simulink model "ulise_internal_v0"  (R2025b)
settings: Solver=FixedStepAuto  StartTime=0.0  StopTime=SimSetup.K - 1  FixedStep=1  RelTol=1e-3
InitFcn:
  | InitFcn_ULISE
model workspace (MAT data in the model file):
  Something = 3
undefined symbols (not defined in the file): A, B, C, D, G, H, Q, R, Sigma, SimSetup, U1, U2, V, V1, V2, x0
libraries: dspinverses x1
settings Model: Creator=savan  LastModifiedBy=daniellawson
settings DebuggingCC: AlgebraicLoopMsg=none

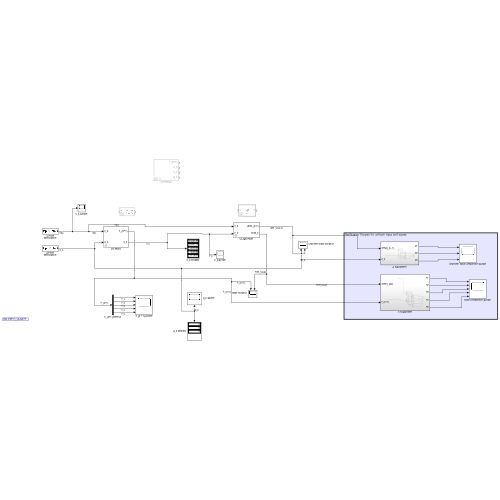
[thumbnail: Simulink's stored preview of the top-level diagram]
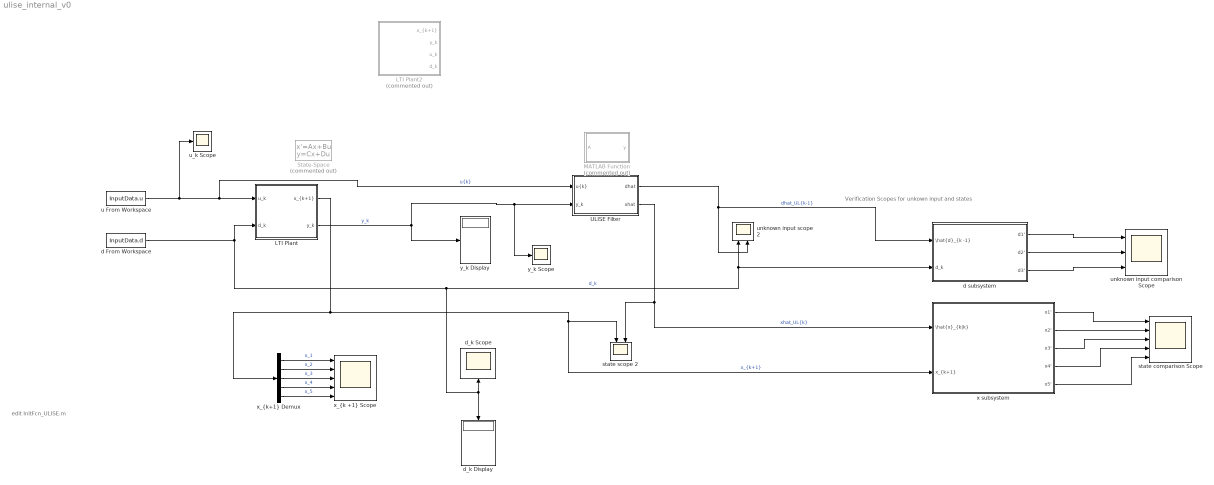
== system ulise_internal_v0 ==
  note: edit InitFcn_ULISE.m
  note: Verification Scopes for unkown input and states
  " u From Workspace" : FromWorkspace  VariableName=InputData.u  SampleTime=SimSetup.Ts  Interpolate=off  OutputAfterFinalValue=Holding final value
  LTI Plant : Subsystem  mask{x0=x0, Ts=SimSetup.Ts}
      mask prompts: x0 "Initial states x[0]:"; Ts "Sample Time (-1 for Inherited):"
      mask help:
      | Simulate the states and measurements of a discrete-time, time-invariant linear system of the form
      |
      | x[k+1] = Ax[k] + Bu[k] + Gd[k]
      | y[k] = Cx[k] + Du[k] + Hd[k].
      mask DialogControl DescGroupVar Prompt: Plant
      mask DialogControl InitialConditions Prompt: Initial Conditions
      mask Display:
      | port_label('input', 1, 'u_k');
      | port_label('input', 2, 'd_k');
      | port_label('output', 1, 'x_{k+1}');
      | port_label('output', 2, 'y_k');
  LTI Plant2 : Subsystem  Commented=on  mask{x0=x0, Ts=SimSetup.Ts}
      mask prompts: x0 "Initial states x[0]:"; Ts "Sample Time (-1 for Inherited):"
      mask help: Simulate the states and measurements of a discrete-time, time-invariant linear system. The user-defined known and unknown inputs are also returned.
      mask DialogControl DescGroupVar Prompt: Plant
      mask DialogControl InitialConditions Prompt: Initial Conditions
      mask Display:
      | port_label('output', 1, 'x_{k+1}');
      | port_label('output', 2, 'y_k');
      | port_label('output', 3, 'u_k');
      | port_label('output', 4, 'd_k');
  MATLAB Function : MATLAB Function  Commented=on  TreatAsAtomicUnit=on
  State-Space : StateSpace  Commented=on  InitialCondition=0
  ULISE Filter : Subsystem  mask{Ts=-1}
      mask prompts: Ts "Sample time (-1 for Inherited):"
      mask help: Estimates the states and unknown inputs of a discrete-time, time-invariant linear system. The states are estimated with a zero-step delay, while the unknown inputs are estimated with a one-step delay.
      mask DialogControl DescGroupVar Prompt: ULISE Filter
      mask Display:
      | port_label('input', 1, 'u_k');
      | port_label('input', 2, 'y_k');
      | port_label('output', 1, 'dhat_{k-1}');
      | port_label('output', 2, 'xhat_k');
  d From Workspace : FromWorkspace  VariableName=InputData.d  SampleTime=SimSetup.Ts  Interpolate=off  OutputAfterFinalValue=Holding final value
  d subsystem : Subsystem
  d_k Display : Display
  d_k Scope : Scope
      settings: ActiveDisplayYMinimum=-3.75  ActiveDisplayYMaximum=3.75
  state comparison Scope : Scope  NumInputPorts=5
      settings: ActiveDisplayString=5  ActiveDisplayYMinimum=-0.034557973978604738  ActiveDisplayYMaximum=0.034947051285830096  YLabel=x_5  DataLoggingVariableName=ScopeData7
  state scope 2 : Scope  NumInputPorts=2
      settings: ActiveDisplayYMinimum=-1  ActiveDisplayYMaximum=1  DataLoggingVariableName=ScopeData9
  u_k Scope : Scope
      settings: ActiveDisplayYMinimum=-0.9712898122759519  ActiveDisplayYMaximum=0.99793476405615489  DataLoggingVariableName=ScopeData2
  unknown input comparison Scope : Scope  NumInputPorts=3
      settings: ActiveDisplayString=3  ActiveDisplayYMinimum=-5.0027563624884559  ActiveDisplayYMaximum=4.879938565566035  YLabel=d_3  DataLoggingVariableName=ScopeData8
  unknown input scope 2 : Scope  NumInputPorts=2
      settings: ActiveDisplayYMinimum=-3.75  ActiveDisplayYMaximum=3.75  DataLoggingVariableName=ScopeData10
  x subsystem : Subsystem
  "x_{k +1} Scope" : Scope  NumInputPorts=5
      settings: Title=%<SignalLabel> vs. time  ActiveDisplayYMinimum=-3.2438704596017818  ActiveDisplayYMaximum=10.248440676542884  YLabel=x_1  DataLoggingVariableName=ScopeData4
  "x_{k+1} Demux" : Demux  Outputs=size(A,1)
  y_k Display : Display
  y_k Scope : Scope
      settings: ActiveDisplayYMinimum=-7.4398331257700985  ActiveDisplayYMaximum=13.958793119448332
  wires:
  x subsystem/1(x1') -> state comparison Scope/1
  x subsystem/2(x2') -> state comparison Scope/2
  x subsystem/3(x3') -> state comparison Scope/3
  x subsystem/4(x4') -> state comparison Scope/4
  x subsystem/5(x5') -> state comparison Scope/5
  d subsystem/1(d1') -> unknown input comparison Scope/1
  d subsystem/2(d2') -> unknown input comparison Scope/2
  d subsystem/3(d3') -> unknown input comparison Scope/3
  ULISE Filter/2(xhat) -> x subsystem/1("\\hat{x}_{k|k}"), state scope 2/2  "xhat_UL{k}"
  ULISE Filter/1(dhat) -> d subsystem/1("\\hat{d}_{k -1}"), unknown input scope 2/2  "dhat_UL{k-1}"
  " u From Workspace"/1 -> u_k Scope/1, LTI Plant/1(u_k), ULISE Filter/1("u{k}")  "u{k}"
  LTI Plant/2(y_k) -> y_k Display/1, y_k Scope/1, ULISE Filter/2(y_k)  "y_k"
  "x_{k+1} Demux"/1 -> "x_{k +1} Scope"/1  "x_1"
  "x_{k+1} Demux"/2 -> "x_{k +1} Scope"/2  "x_2"
  "x_{k+1} Demux"/4 -> "x_{k +1} Scope"/4  "x_4"
  "x_{k+1} Demux"/3 -> "x_{k +1} Scope"/3  "x_3"
  "x_{k+1} Demux"/5 -> "x_{k +1} Scope"/5  "x_5"
  LTI Plant/1("x_{k+1}") -> "x_{k+1} Demux"/1, x subsystem/2("x_{k+1}"), state scope 2/1  "x_{k+1}"
  d From Workspace/1 -> d_k Scope/1, d_k Display/1, d subsystem/2(d_k), unknown input scope 2/1, LTI Plant/2(d_k)  "d_k"

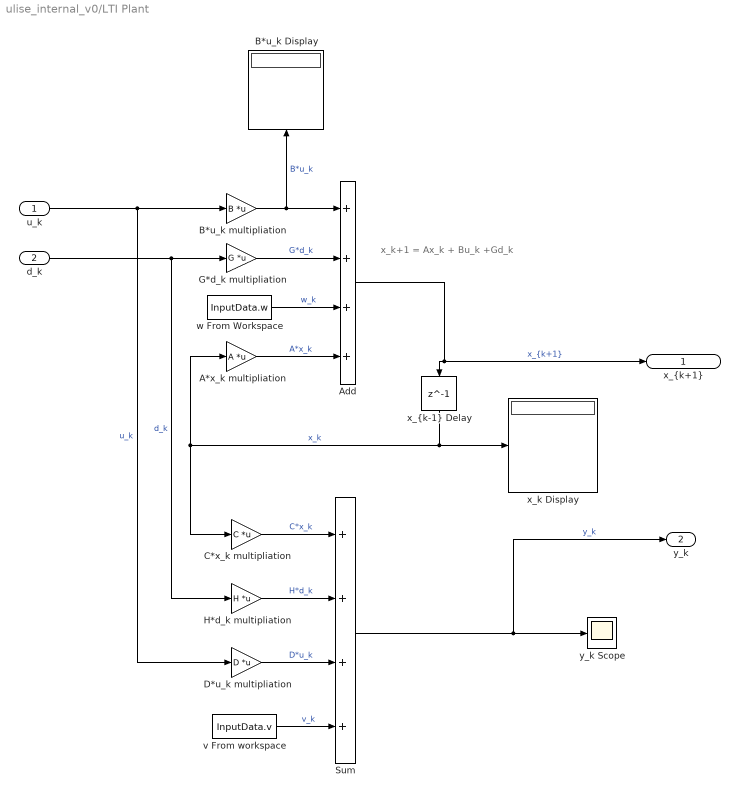
== system ulise_internal_v0/LTI Plant ==
  note: x_k+1 = Ax_k + Bu_k +Gd_k
  u_k : Inport
  d_k : Inport  Port=2
  A*x_k multipliation : Gain  Gain=A  Multiplication=Matrix(K*u)
  Add : Sum  Inputs=++++
  B*u_k Display : Display
  B*u_k multipliation : Gain  Gain=B  Multiplication=Matrix(K*u)
  C*x_k multipliation : Gain  Gain=C  Multiplication=Matrix(K*u)
  D*u_k multipliation : Gain  Gain=D  Multiplication=Matrix(K*u)
  G*d_k multipliation : Gain  Gain=G  Multiplication=Matrix(K*u)
  H*d_k multipliation : Gain  Gain=H  Multiplication=Matrix(K*u)
  Sum : Sum  Inputs=++++
  v From workspace : FromWorkspace  VariableName=InputData.v  SampleTime=SimSetup.Ts  Interpolate=off  OutputAfterFinalValue=Holding final value
  w From Workspace : FromWorkspace  VariableName=InputData.w  SampleTime=SimSetup.Ts  Interpolate=off  OutputAfterFinalValue=Holding final value
  x_k Display : Display
  "x_{k-1} Delay" : Delay  DelayLength=1  InitialCondition=x0
  y_k Scope : Scope
      settings: ActiveDisplayYMinimum=-7.0592065430833646  ActiveDisplayYMaximum=14.061490045979077  DataLoggingVariableName=ScopeData5
  "x_{k+1}" : Outport
  y_k : Outport  Port=2
  wires:
  D*u_k multipliation/1 -> Sum/3  "D*u_k"
  v From workspace/1 -> Sum/4  "v_k"
  H*d_k multipliation/1 -> Sum/2  "H*d_k"
  G*d_k multipliation/1 -> Add/2  "G*d_k"
  C*x_k multipliation/1 -> Sum/1  "C*x_k"
  Sum/1 -> y_k/1, y_k Scope/1  "y_k"
  "x_{k-1} Delay"/1 -> A*x_k multipliation/1, C*x_k multipliation/1, x_k Display/1  "x_k"
  w From Workspace/1 -> Add/3  "w_k"
  B*u_k multipliation/1 -> Add/1, B*u_k Display/1  "B*u_k"
  Add/1 -> "x_{k+1}"/1, "x_{k-1} Delay"/1  "x_{k+1}"
  A*x_k multipliation/1 -> Add/4  "A*x_k"
  d_k/1 -> H*d_k multipliation/1, G*d_k multipliation/1  "d_k"
  u_k/1 -> D*u_k multipliation/1, B*u_k multipliation/1  "u_k"

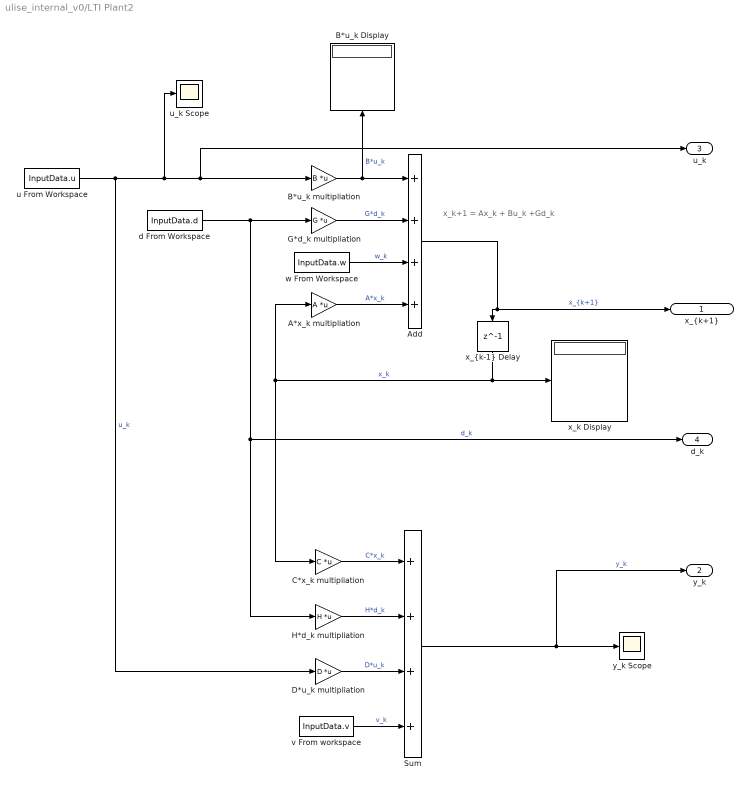
== system ulise_internal_v0/LTI Plant2 ==
  note: x_k+1 = Ax_k + Bu_k +Gd_k
  " u From Workspace" : FromWorkspace  VariableName=InputData.u  SampleTime=SimSetup.Ts  Interpolate=off  OutputAfterFinalValue=Holding final value
  A*x_k multipliation : Gain  Gain=A  Multiplication=Matrix(K*u)
  Add : Sum  Inputs=++++
  B*u_k Display : Display
  B*u_k multipliation : Gain  Gain=B  Multiplication=Matrix(K*u)
  C*x_k multipliation : Gain  Gain=C  Multiplication=Matrix(K*u)
  D*u_k multipliation : Gain  Gain=D  Multiplication=Matrix(K*u)
  G*d_k multipliation : Gain  Gain=G  Multiplication=Matrix(K*u)
  H*d_k multipliation : Gain  Gain=H  Multiplication=Matrix(K*u)
  Sum : Sum  Inputs=++++
  d From Workspace : FromWorkspace  VariableName=InputData.d  SampleTime=SimSetup.Ts  Interpolate=off  OutputAfterFinalValue=Holding final value
  u_k Scope : Scope
      settings: ActiveDisplayYMinimum=-0.9712898122759519  ActiveDisplayYMaximum=0.99793476405615489  DataLoggingVariableName=ScopeData6
  v From workspace : FromWorkspace  VariableName=InputData.v  SampleTime=SimSetup.Ts  Interpolate=off  OutputAfterFinalValue=Holding final value
  w From Workspace : FromWorkspace  VariableName=InputData.w  SampleTime=SimSetup.Ts  Interpolate=off  OutputAfterFinalValue=Holding final value
  x_k Display : Display
  "x_{k-1} Delay" : Delay  DelayLength=1  InitialCondition=x0
  y_k Scope : Scope
      settings: ActiveDisplayYMinimum=-7.0592065430833646  ActiveDisplayYMaximum=14.061490045979077  DataLoggingVariableName=ScopeData5
  "x_{k+1}" : Outport
  y_k : Outport  Port=2
  u_k : Outport  Port=3
  d_k : Outport  Port=4
  wires:
  D*u_k multipliation/1 -> Sum/3  "D*u_k"
  v From workspace/1 -> Sum/4  "v_k"
  " u From Workspace"/1 -> u_k Scope/1, u_k/1, B*u_k multipliation/1, D*u_k multipliation/1  "u_k"
  H*d_k multipliation/1 -> Sum/2  "H*d_k"
  G*d_k multipliation/1 -> Add/2  "G*d_k"
  C*x_k multipliation/1 -> Sum/1  "C*x_k"
  Sum/1 -> y_k/1, y_k Scope/1  "y_k"
  "x_{k-1} Delay"/1 -> A*x_k multipliation/1, C*x_k multipliation/1, x_k Display/1  "x_k"
  w From Workspace/1 -> Add/3  "w_k"
  d From Workspace/1 -> H*d_k multipliation/1, d_k/1, G*d_k multipliation/1  "d_k"
  B*u_k multipliation/1 -> Add/1, B*u_k Display/1  "B*u_k"
  Add/1 -> "x_{k+1}"/1, "x_{k-1} Delay"/1  "x_{k+1}"
  A*x_k multipliation/1 -> Add/4  "A*x_k"

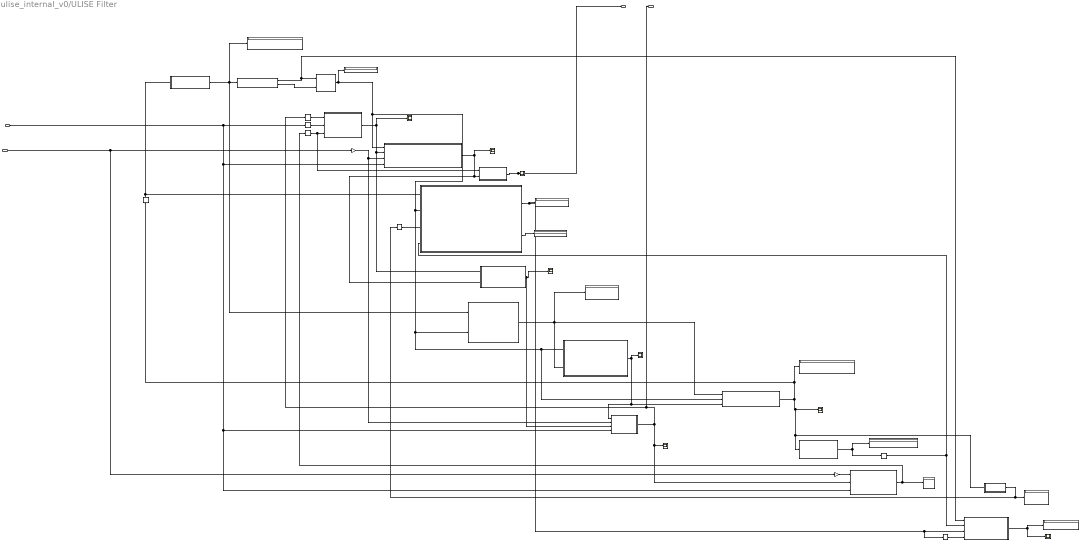
== system ulise_internal_v0/ULISE Filter ==
  note: estimate d1
  "u{k}" : Inport
  y_k : Inport  Port=2
  "Compute L_{k}" : Subsystem
  "Compute M_UL{k}" : Subsystem
  "Compute P_tilde_UL{k}" : Subsystem
  "Compute Pd12_{k-1} and Pxd2_{k-1}" : Subsystem
  "Compute Pd1_{k}" : Subsystem
  "Compute Pd2_{k-1}" : Subsystem
  "Compute Pd_{k -1}" : Subsystem
  "Compute Px_star_{k}" : Subsystem
  "Compute Px_{k | k}" : Subsystem
  "Compute Pxd1_{k}" : Subsystem
  "Compute measurement update, xhat_{k | k}" : Subsystem
  "Compute observable unknown input, dhat1_{k}" : Subsystem
  "Compute state prediction, xhat_{k | k-1} " : Subsystem
  "Compute time updated state, xhat_star_{k | k}" : Subsystem
  "Compute unknown input, dhat_{k-1}" : Subsystem
  "Compute unobservable unknown input, dhat2_{k-1}" : Subsystem
  "L_UL{k} Scope" : Scope
      settings: DataLoggingVariableName=ScopeData15
  "M_UL{k} Display" : Display
  "P_tilde{k} Display" : Display
  "Pd12_UL{k-1} Display" : Display
  "Pd12_UL{k-1} Transpose" : Math  Operator=transpose
  "Pd1_UL{k} Delay" : Delay  DelayLength=1
  "Pd1_UL{k} Display" : Display
  "Pd_UL{k-1} Display" : Display
  "Pd_UL{k-1} Scope" : Scope
      settings: ActiveDisplayYMinimum=-2.8647454783400574  ActiveDisplayYMaximum=2.0010614488413259  DataLoggingVariableName=ScopeData18
  "Px_UL{k} Delay" : Delay  DelayLength=1
  "Px_UL{k} Display" : Display
  "Px_UL{k} Scope" : Scope
      settings: ActiveDisplayYMinimum=-1  ActiveDisplayYMaximum=1  DataLoggingVariableName=ScopeData17
  "Px_star_UL{k} Display" : Display
  "Pxd1_UL{k} Delay" : Delay  DelayLength=1
  "Pxd1_UL{k} Display" : Display
  "Pxd2_UL{k-1} Display" : Display
  "dhat 1_UL{k} Display" : Display
  "dhat1_UL{k} Delay" : Delay  DelayLength=1
  "dhat2_UL{k-1} Scope" : Scope
      settings: DataLoggingVariableName=ScopeData12
  "dhat{k-1} Scope" : Scope
      settings: ActiveDisplayYMinimum=-1  ActiveDisplayYMaximum=1  DataLoggingVariableName=ScopeData13
  left-multiply y_k by T1 : Gain  Gain=(U1' - U1'*R*U2*inv(U2'*R*U2)*U2')  Multiplication=Matrix(K*u)
  "left-multiply y_k by T2 " : Gain  Gain=U2'  Multiplication=Matrix(K*u)
  "u{k} Delay" : Delay  DelayLength=1
  "xhat_UL{k} Delay" : Delay  DelayLength=1
  "xhat_UL{k} Scope" : Scope
      settings: ActiveDisplayYMinimum=-9.9265677386173241  ActiveDisplayYMaximum=15.803450039955713  DataLoggingVariableName=ScopeData16
  "xhat_p_UL{k} Scope" : Scope
      settings: DataLoggingVariableName=ScopeData11
  "xhat_star_UL{k} Scope" : Scope
      settings: DataLoggingVariableName=ScopeData14
  dhat : Outport
  xhat : Outport  Port=2
  wires:
  "Pd1_UL{k} Delay"/1 -> "Compute Pd12_{k-1} and Pxd2_{k-1}"/4("Pd1_UL{k-1}"), "Compute Pd_{k -1}"/2("Pd1_UL{k-1}")  "Pd1_UL{k-1}"
  "Px_UL{k} Delay"/1 -> "Compute P_tilde_UL{k}"/1("Px_UL{k-1}"), "Compute Pd12_{k-1} and Pxd2_{k-1}"/1("Px_UL{k-1}")  "Px_UL{k-1}"
  "left-multiply y_k by T2 "/1 -> "Compute measurement update, xhat_{k | k}"/2("z2{k}"), "Compute unobservable unknown input, dhat2_{k-1}"/3("z2{k}")  "z2{k}"
  "u{k}"/1 -> "u{k} Delay"/1, "Compute unobservable unknown input, dhat2_{k-1}"/4("u{k-1}"), "Compute observable unknown input, dhat1_{k}"/3("u{k-1}"), "Compute measurement update, xhat_{k | k}"/4("u{k-1}")  "u_k"
  y_k/1 -> left-multiply y_k by T1/1, "left-multiply y_k by T2 "/1  "y_k"
  "dhat1_UL{k} Delay"/1 -> "Compute unknown input, dhat_{k-1}"/1("dhat1_UL{k-1}"), "Compute state prediction, xhat_{k | k-1} "/3("dhat1_UL{k-1}")  "dhat1_UL{k-1}"
  "Compute state prediction, xhat_{k | k-1} "/1("xhat_p_UL{k}") -> "xhat_p_UL{k} Scope"/1, "Compute time updated state, xhat_star_{k | k}"/1("xhat_p_UL{k}"), "Compute unobservable unknown input, dhat2_{k-1}"/2("xhat_p_UL{k}")  "xhat_p_UL{k}"
  "xhat_UL{k} Delay"/1 -> "Compute state prediction, xhat_{k | k-1} "/1("xhat_UL{k-1}")  "xhat_UL{k-1}"
  "u{k} Delay"/1 -> "Compute state prediction, xhat_{k | k-1} "/2("u{k-1}")  "u{k-1}"
  "Compute unobservable unknown input, dhat2_{k-1}"/1("dhat2_UL{k-1}") -> "dhat2_UL{k-1} Scope"/1, "Compute unknown input, dhat_{k-1}"/2("dhat2_UL{k-1}"), "Compute time updated state, xhat_star_{k | k}"/2("dhat2_UL{k-1}")  "dhat2_UL{k-1}"
  "Compute unknown input, dhat_{k-1}"/1("dhat_UL{k-1}") -> dhat/1, "dhat{k-1} Scope"/1
  "Compute time updated state, xhat_star_{k | k}"/1("xhat_star_UL{k}") -> "xhat_star_UL{k} Scope"/1, "Compute measurement update, xhat_{k | k}"/3("xhat_star_UL{k}")  "xhat_star_UL{k}"
  "Compute measurement update, xhat_{k | k}"/1("xhat_UL{k}") -> xhat/1, "xhat_UL{k} Delay"/1, "xhat_UL{k} Scope"/1, "Compute observable unknown input, dhat1_{k}"/2("xhat_UL{k}")  "xhat_UL{k}"
  "Compute observable unknown input, dhat1_{k}"/1("dhat1_UL{k}") -> "dhat 1_UL{k} Display"/1, "dhat1_UL{k} Delay"/1  "dhat1_UL{k}"
  "Compute Pxd1_{k}"/1("Pxd1_UL{k}") -> "Pxd1_UL{k} Delay"/1, "Pxd1_UL{k} Display"/1  "Pxd1_UL{k}"
  "Compute Pd_{k -1}"/1("Pd_UL{k-1}") -> "Pd_UL{k-1} Display"/1, "Pd_UL{k-1} Scope"/1  "Pd_UL{k-1}"
  "Pd12_UL{k-1} Transpose"/1 -> "Compute Pd_{k -1}"/4("(Pd12_UL{k-1})^T")  "(Pd12_UL{k-1})^T"
  "Compute Pd1_{k}"/1("Pd1_UL{k}") -> "Pd1_UL{k} Delay"/1, "Pd1_UL{k} Display"/1  "Pd1_UL{k}"
  "Compute Px_{k | k}"/1("Px_UL{k}") -> "Px_UL{k} Delay"/1, "Px_UL{k} Display"/1, "Px_UL{k} Scope"/1, "Compute Pd1_{k}"/1("Px_UL{k}"), "Compute Pxd1_{k}"/1("Px_UL{k}")  "Px_UL{k}"
  "Compute L_{k}"/1("L_UL{k}") -> "L_UL{k} Scope"/1, "Compute Px_{k | k}"/3("L_UL{k}"), "Compute measurement update, xhat_{k | k}"/1("L_UL{k}")  "L_UL{k}"
  "Compute Px_star_{k}"/1("Px_star_UL{k}") -> "Compute L_{k}"/2("Px_star_UL{k}"), "Compute Px_{k | k}"/1("Px_star_UL{k}"), "Px_star_UL{k} Display"/1  "Px_star_UL{k}"
  "Compute Pd12_{k-1} and Pxd2_{k-1}"/1("Pd12_UL{k-1}") -> "Pd12_UL{k-1} Display"/1, "Compute Pd_{k -1}"/3("Pd12_UL{k-1}"), "Pd12_UL{k-1} Transpose"/1  "Pd12_UL{k-1}"
  "Pxd1_UL{k} Delay"/1 -> "Compute Pd12_{k-1} and Pxd2_{k-1}"/3("Pxd1_UL{k-1}")  "Pxd1_UL{k-1}"
  "Compute Pd12_{k-1} and Pxd2_{k-1}"/2("Pxd2_UL{k-1}") -> "Pxd2_UL{k-1} Display"/1  "Pxd2_UL{k-1}"
  "Compute Pd2_{k-1}"/1("Pd2_UL{k-1}") -> "Compute Pd_{k -1}"/1("Pd2_UL{k-1}"), "Compute M_UL{k}"/1("Pd2_UL{k-1}")  "Pd2_UL{k-1}"
  "Compute P_tilde_UL{k}"/1("P_tilde_UL{k}") -> "Compute Px_star_{k}"/1("P_tilde_UL{k}"), "P_tilde{k} Display"/1, "Compute Pd2_{k-1}"/1("P_tilde_UL{k}")
  "Compute M_UL{k}"/1("M_UL{k}") -> "Compute unobservable unknown input, dhat2_{k-1}"/1("M_UL{k}"), "Compute L_{k}"/1("M_UL{k}"), "Compute Px_{k | k}"/2("M_UL{k}"), "Compute Px_star_{k}"/2("M_UL{k}"), "Compute Pd12_{k-1} and Pxd2_{k-1}"/2("M_UL{k}"), "M_UL{k} Display"/1  "M_UL{k}"
  "Compute Pd2_{k-1}"/2("G2^T*C2^T*inv(R2_tilde_UL{k})") -> "Compute M_UL{k}"/2("G2^T*C2^T*inv(R2_tilde_UL{k})")  "G2^T*C2^T*inv(R2_tilde_UL{k})"
  left-multiply y_k by T1/1 -> "Compute observable unknown input, dhat1_{k}"/1("z1{k}")  "z1{k}"

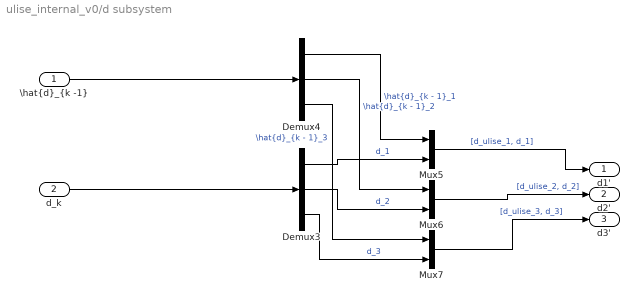
== system ulise_internal_v0/d subsystem ==
  "\\hat{d}_{k -1}" : Inport
  d_k : Inport  Port=2
  Demux3 : Demux  Outputs=size(G,2)
  Demux4 : Demux  Outputs=size(G,2)
  Mux5 : Mux  Inputs=2
  Mux6 : Mux  Inputs=2
  Mux7 : Mux  Inputs=2
  d1' : Outport
  d2' : Outport  Port=2
  d3' : Outport  Port=3
  wires:
  Mux6/1 -> d2'/1  "[d_ulise_2, d_2]"
  d_k/1 -> Demux3/1
  Mux7/1 -> d3'/1  "[d_ulise_3, d_3]"
  Demux3/3 -> Mux7/2  "d_3"
  Demux4/1 -> Mux5/1  "\\hat{d}_{k - 1}_1"
  Demux4/2 -> Mux6/1  "\\hat{d}_{k - 1}_2"
  "\\hat{d}_{k -1}"/1 -> Demux4/1
  Mux5/1 -> d1'/1  "[d_ulise_1, d_1]"
  Demux3/2 -> Mux6/2  "d_2"
  Demux3/1 -> Mux5/2  "d_1"
  Demux4/3 -> Mux7/1  "\\hat{d}_{k - 1}_3"

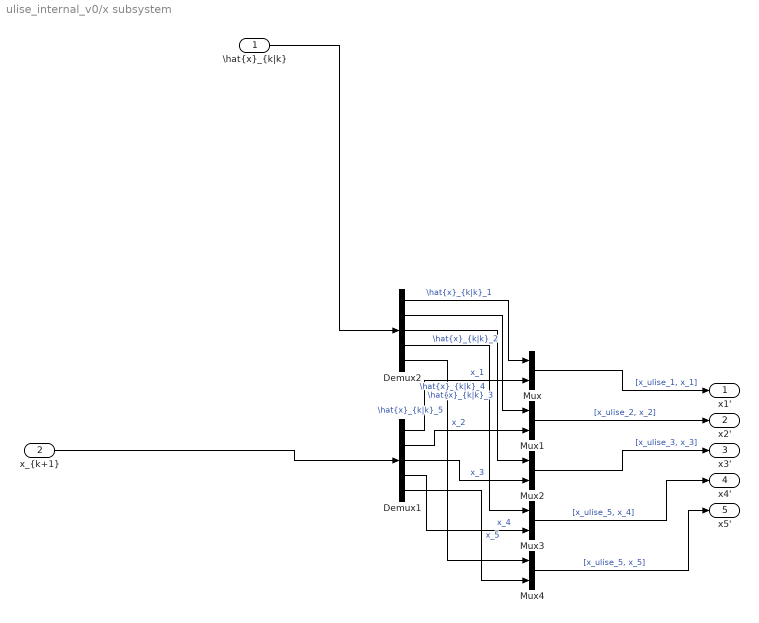
== system ulise_internal_v0/x subsystem ==
  "\\hat{x}_{k|k}" : Inport
  "x_{k+1}" : Inport  Port=2
  Demux1 : Demux  Outputs=size(A,1)
  Demux2 : Demux  Outputs=size(A,1)
  Mux{,1..4} (5 alike) : Mux  Inputs=2
  x1' : Outport
  x2' : Outport  Port=2
  x3' : Outport  Port=3
  x4' : Outport  Port=4
  x5' : Outport  Port=5
  wires:
  Mux/1 -> x1'/1  "[x_ulise_1, x_1]"
  "\\hat{x}_{k|k}"/1 -> Demux2/1
  Mux4/1 -> x5'/1  "[x_ulise_5, x_5]"
  Mux2/1 -> x3'/1  "[x_ulise_3, x_3]"
  Demux1/4 -> Mux3/2  "x_4"
  Mux3/1 -> x4'/1  "[x_ulise_5, x_4]"
  Mux1/1 -> x2'/1  "[x_ulise_2, x_2]"
  Demux1/2 -> Mux1/2  "x_2"
  Demux1/3 -> Mux2/2  "x_3"
  Demux2/5 -> Mux4/1  "\\hat{x}_{k|k}_5"
  Demux2/1 -> Mux/1  "\\hat{x}_{k|k}_1"
  Demux2/4 -> Mux3/1  "\\hat{x}_{k|k}_4"
  Demux2/2 -> Mux1/1  "\\hat{x}_{k|k}_2"
  "x_{k+1}"/1 -> Demux1/1
  Demux1/5 -> Mux4/2  "x_5"
  Demux2/3 -> Mux2/1  "\\hat{x}_{k|k}_3"
  Demux1/1 -> Mux/2  "x_1"

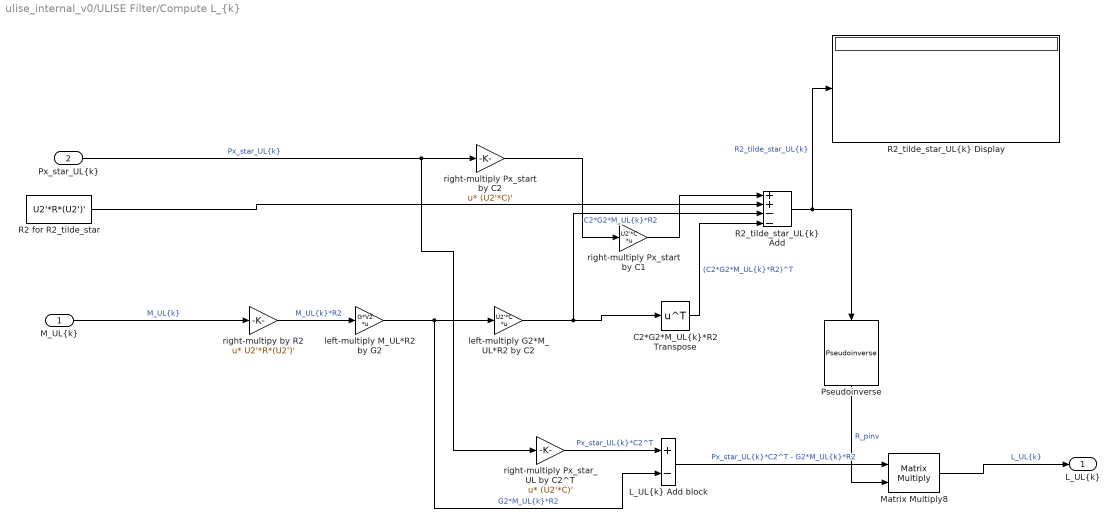
== system ulise_internal_v0/ULISE Filter/Compute L_{k} ==
  "M_UL{k}" : Inport
  "Px_star_UL{k}" : Inport  Port=2
  " R2 for R2_tilde_star" : Constant  Value=U2'*R*(U2')'  VectorParams1D=off
  "C2*G2*M_UL{k}*R2 Transpose" : Math  Operator=transpose
  "L_UL{k} Add block" : Sum  Inputs=+-
  Matrix Multiply8 : Product  Multiplication=Matrix(*)
  Pseudoinverse : dspinverses/Pseudoinverse  wanterr=off  SimulateUsing=Interpreted execution
  "R2_tilde_star_UL{k} Add" : Sum  Inputs=++--
  "R2_tilde_star_UL{k} Display" : Display
  left-multiply G2*M_UL*R2 by C2 : Gain  Gain=U2'*C  Multiplication=Matrix(K*u)
  left-multiply M_UL*R2 by G2 : Gain  Gain=G*V2  Multiplication=Matrix(K*u)
  "right-multiply Px_star_UL by C2^T " : Gain  Gain=(U2'*C)'  Multiplication=Matrix(u*K)
  right-multiply Px_start by C1 : Gain  Gain=U2'*C  Multiplication=Matrix(K*u)
  right-multiply Px_start by C2 : Gain  Gain=(U2'*C)'  Multiplication=Matrix(u*K)
  right-multipy by R2 : Gain  Gain=U2'*R*(U2')'  Multiplication=Matrix(u*K)
  "L_UL{k}" : Outport
  wires:
  right-multipy by R2/1 -> left-multiply M_UL*R2 by G2/1  "M_UL{k}*R2"
  "Px_star_UL{k}"/1 -> right-multiply Px_start by C2/1, "right-multiply Px_star_UL by C2^T "/1  "Px_star_UL{k}"
  Matrix Multiply8/1 -> "L_UL{k}"/1  "L_UL{k}"
  Pseudoinverse/1 -> Matrix Multiply8/2  "R_pinv"
  "right-multiply Px_star_UL by C2^T "/1 -> "L_UL{k} Add block"/1  "Px_star_UL{k}*C2^T"
  right-multiply Px_start by C2/1 -> right-multiply Px_start by C1/1
  left-multiply M_UL*R2 by G2/1 -> "L_UL{k} Add block"/2, left-multiply G2*M_UL*R2 by C2/1  "G2*M_UL{k}*R2"
  "R2_tilde_star_UL{k} Add"/1 -> "R2_tilde_star_UL{k} Display"/1, Pseudoinverse/1  "R2_tilde_star_UL{k}"
  left-multiply G2*M_UL*R2 by C2/1 -> "R2_tilde_star_UL{k} Add"/3, "C2*G2*M_UL{k}*R2 Transpose"/1  "C2*G2*M_UL{k}*R2"
  "L_UL{k} Add block"/1 -> Matrix Multiply8/1  "Px_star_UL{k}*C2^T - G2*M_UL{k}*R2"
  " R2 for R2_tilde_star"/1 -> "R2_tilde_star_UL{k} Add"/2
  "M_UL{k}"/1 -> right-multipy by R2/1  "M_UL{k}"
  right-multiply Px_start by C1/1 -> "R2_tilde_star_UL{k} Add"/1
  "C2*G2*M_UL{k}*R2 Transpose"/1 -> "R2_tilde_star_UL{k} Add"/4  "(C2*G2*M_UL{k}*R2)^T"

== system ulise_internal_v0/ULISE Filter/Compute M_UL{k} ==
  "Pd2_UL{k-1}" : Inport
  "G2^T*C2^T*inv(R2_tilde_UL{k})" : Inport  Port=2
  Matrix Multiply : Product  Multiplication=Matrix(*)
  "M_UL{k}" : Outport
  wires:
  "G2^T*C2^T*inv(R2_tilde_UL{k})"/1 -> Matrix Multiply/2  "G2^T*C2^T*inv(R2_tilde_UL{k})"
  Matrix Multiply/1 -> "M_UL{k}"/1  "M_UL{k}"
  "Pd2_UL{k-1}"/1 -> Matrix Multiply/1  "Pd2_UL{k-1}"

== system ulise_internal_v0/ULISE Filter/Compute P_tilde_UL{k} ==
  "Px_UL{k-1}" : Inport
  Add Qhat : Sum
  Qhat : Constant  Value=G*V1*pinv(Sigma)*((U1' - U1'*R*U2*inv(U2'*R*U2)*U2')*R*(U1' - U1'*R*U2*inv(U2'*R*U2)*U2')')*pinv(Sigma)'*(G*V1)' + Q  VectorParams1D=off
  left-multiply by Ahat : Gain  Gain=A - G*V1*pinv(Sigma)*((U1' - U1'*R*U2*inv(U2'*R*U2)*U2')*C)  Multiplication=Matrix(K*u)
  right-multiply by Ahat^T : Gain  Gain=(A - G*V1*pinv(Sigma)*((U1' - U1'*R*U2*inv(U2'*R*U2)*U2')*C))'  Multiplication=Matrix(u*K)
  "P_tilde_UL{k}" : Outport
  wires:
  Add Qhat/1 -> "P_tilde_UL{k}"/1  "P_tilde_UL{k}"
  "Px_UL{k-1}"/1 -> right-multiply by Ahat^T/1  "Px_UL{k-1}"
  right-multiply by Ahat^T/1 -> left-multiply by Ahat/1  "Px_UL{k-1}*Ahat^T"
  left-multiply by Ahat/1 -> Add Qhat/1  "Ahat*Px_UL{k-1}*Ahat^T"
  Qhat/1 -> Add Qhat/2  "Qhat"

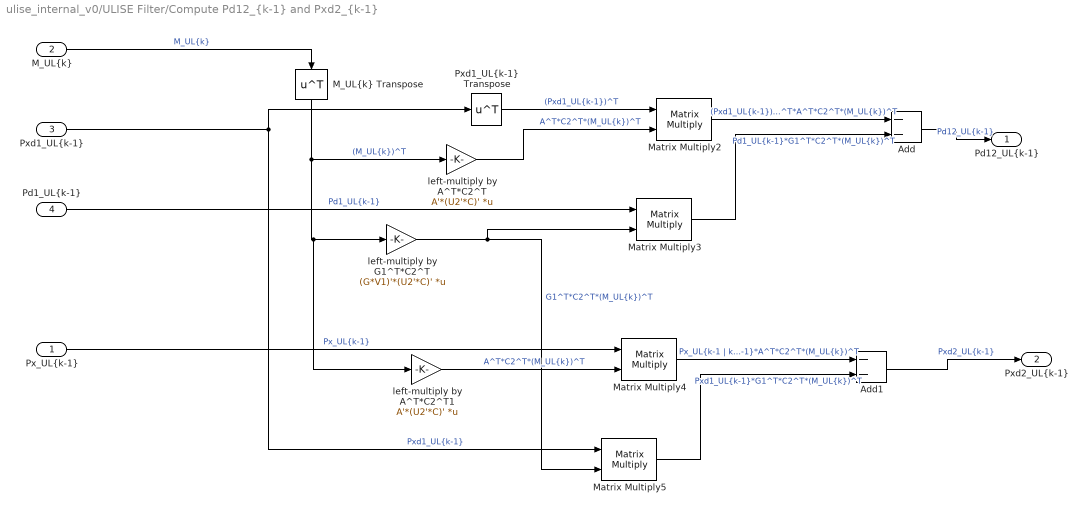
== system ulise_internal_v0/ULISE Filter/Compute Pd12_{k-1} and Pxd2_{k-1} ==
  "Px_UL{k-1}" : Inport
  "M_UL{k}" : Inport  Port=2
  "Pxd1_UL{k-1}" : Inport  Port=3
  "Pd1_UL{k-1}" : Inport  Port=4
  Add : Sum  Inputs=--
  Add1 : Sum  Inputs=--
  "M_UL{k} Transpose" : Math  Operator=transpose
  Matrix Multiply{2..5} (4 alike) : Product  Multiplication=Matrix(*)
  "Pxd1_UL{k-1} Transpose" : Math  Operator=transpose
  left-multiply by A^T*C2^T : Gain  Gain=A'*(U2'*C)'  Multiplication=Matrix(K*u)
  left-multiply by A^T*C2^T1 : Gain  Gain=A'*(U2'*C)'  Multiplication=Matrix(K*u)
  left-multiply by G1^T*C2^T : Gain  Gain=(G*V1)'*(U2'*C)'  Multiplication=Matrix(K*u)
  "Pd12_UL{k-1}" : Outport
  "Pxd2_UL{k-1}" : Outport  Port=2
  wires:
  Add1/1 -> "Pxd2_UL{k-1}"/1  "Pxd2_UL{k-1}"
  left-multiply by A^T*C2^T/1 -> Matrix Multiply2/2  "A^T*C2^T*(M_UL{k})^T"
  Matrix Multiply5/1 -> Add1/2  "Pxd1_UL{k-1}*G1^T*C2^T*(M_UL{k})^T"
  left-multiply by G1^T*C2^T/1 -> Matrix Multiply5/2, Matrix Multiply3/2  "G1^T*C2^T*(M_UL{k})^T"
  left-multiply by A^T*C2^T1/1 -> Matrix Multiply4/2  "A^T*C2^T*(M_UL{k})^T"
  Matrix Multiply3/1 -> Add/2  "Pd1_UL{k-1}*G1^T*C2^T*(M_UL{k})^T"
  "M_UL{k}"/1 -> "M_UL{k} Transpose"/1  "M_UL{k}"
  "Pd1_UL{k-1}"/1 -> Matrix Multiply3/1  "Pd1_UL{k-1}"
  Add/1 -> "Pd12_UL{k-1}"/1  "Pd12_UL{k-1}"
  Matrix Multiply4/1 -> Add1/1  "Px_UL{k-1 | k-1}*A^T*C2^T*(M_UL{k})^T"
  "Px_UL{k-1}"/1 -> Matrix Multiply4/1  "Px_UL{k-1}"
  Matrix Multiply2/1 -> Add/1  "(Pxd1_UL{k-1})^T*A^T*C2^T*(M_UL{k})^T"
  "Pxd1_UL{k-1} Transpose"/1 -> Matrix Multiply2/1  "(Pxd1_UL{k-1})^T"
  "Pxd1_UL{k-1}"/1 -> Matrix Multiply5/1, "Pxd1_UL{k-1} Transpose"/1  "Pxd1_UL{k-1}"
  "M_UL{k} Transpose"/1 -> left-multiply by A^T*C2^T/1, left-multiply by A^T*C2^T1/1, left-multiply by G1^T*C2^T/1  "(M_UL{k})^T"

== system ulise_internal_v0/ULISE Filter/Compute Pd1_{k} ==
  "Px_UL{k}" : Inport
  "R1 " : Constant  Value=(U1' - U1'*R*U2*inv(U2'*R*U2)*U2')*R*(U1' - U1'*R*U2*inv(U2'*R*U2)*U2')'  VectorParams1D=off  SampleTime=SimSetup.Ts
  "R1_tilde_UL{k} Add" : Sum
  "R1_tilde_UL{k} Display" : Display
  "left-multiply Px_UL{k}*C1^T by C1" : Gain  Gain=(U1' - U1'*R*U2*inv(U2'*R*U2)*U2')*C  Multiplication=Matrix(K*u)
  "left-multiply R1_tilde_UL{k}*M1 by M1" : Gain  Gain=pinv(Sigma)  Multiplication=Matrix(K*u)
  "right-multiply Px_UL{k} by C1" : Gain  Gain=((U1' - U1'*R*U2*inv(U2'*R*U2)*U2')*C)'  Multiplication=Matrix(u*K)
  "right-multiply R1_tilde_UL{k} by M1" : Gain  Gain=pinv(Sigma)  Multiplication=Matrix(u*K)
  "Pd1_UL{k}" : Outport
  wires:
  "Px_UL{k}"/1 -> "right-multiply Px_UL{k} by C1"/1
  "right-multiply Px_UL{k} by C1"/1 -> "left-multiply Px_UL{k}*C1^T by C1"/1  "Px_UL{k}*C1^T"
  "right-multiply R1_tilde_UL{k} by M1"/1 -> "left-multiply R1_tilde_UL{k}*M1 by M1"/1  "R1_tilde_UL{k}*M1"
  "left-multiply R1_tilde_UL{k}*M1 by M1"/1 -> "Pd1_UL{k}"/1  "Pd1_UL{k}"
  "left-multiply Px_UL{k}*C1^T by C1"/1 -> "R1_tilde_UL{k} Add"/1  "C1*Px_UL{k}*C1^T"
  "R1_tilde_UL{k} Add"/1 -> "R1_tilde_UL{k} Display"/1, "right-multiply R1_tilde_UL{k} by M1"/1  "R1_tilde_UL{k}"
  "R1 "/1 -> "R1_tilde_UL{k} Add"/2

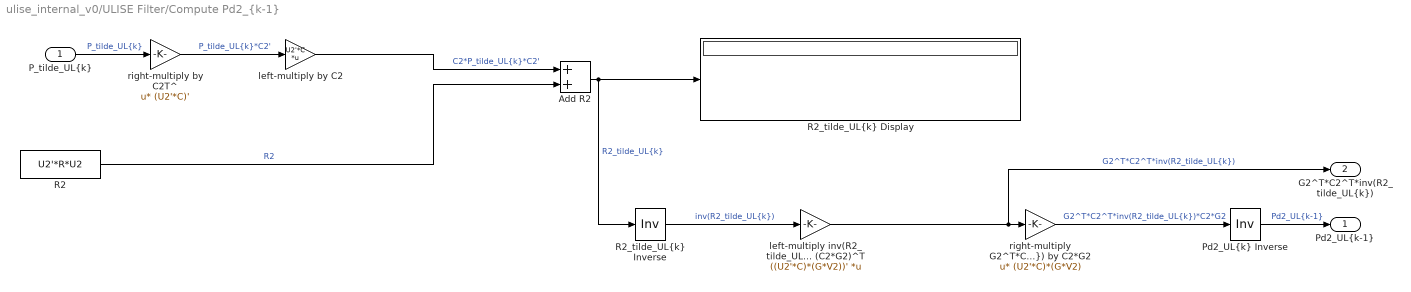
== system ulise_internal_v0/ULISE Filter/Compute Pd2_{k-1} ==
  "P_tilde_UL{k}" : Inport
  Add R2 : Sum
  "Pd2_UL{k} Inverse" : Product  Inputs=/  Multiplication=Matrix(*)
  R2 : Constant  Value=U2'*R*U2  VectorParams1D=off
  "R2_tilde_UL{k} Display" : Display
  "R2_tilde_UL{k} Inverse" : Product  Inputs=/  Multiplication=Matrix(*)
  left-multiply by C2 : Gain  Gain=U2'*C  Multiplication=Matrix(K*u)
  "left-multiply inv(R2_tilde_UL{k}) by (C2*G2)^T " : Gain  Gain=((U2'*C)*(G*V2))'  Multiplication=Matrix(K*u)
  "right-multiply G2^T*C2^T*inv(R2_tilde_UL{k}) by C2*G2" : Gain  Gain=(U2'*C)*(G*V2)  Multiplication=Matrix(u*K)
  right-multiply by C2T^ : Gain  Gain=(U2'*C)'  Multiplication=Matrix(u*K)
  "Pd2_UL{k-1}" : Outport
  "G2^T*C2^T*inv(R2_tilde_UL{k})" : Outport  Port=2
  wires:
  left-multiply by C2/1 -> Add R2/1  "C2*P_tilde_UL{k}*C2'"
  "P_tilde_UL{k}"/1 -> right-multiply by C2T^/1  "P_tilde_UL{k}"
  right-multiply by C2T^/1 -> left-multiply by C2/1  "P_tilde_UL{k}*C2'"
  "right-multiply G2^T*C2^T*inv(R2_tilde_UL{k}) by C2*G2"/1 -> "Pd2_UL{k} Inverse"/1  "G2^T*C2^T*inv(R2_tilde_UL{k})*C2*G2"
  "R2_tilde_UL{k} Inverse"/1 -> "left-multiply inv(R2_tilde_UL{k}) by (C2*G2)^T "/1  "inv(R2_tilde_UL{k})"
  R2/1 -> Add R2/2  "R2"
  "Pd2_UL{k} Inverse"/1 -> "Pd2_UL{k-1}"/1  "Pd2_UL{k-1}"
  Add R2/1 -> "R2_tilde_UL{k} Inverse"/1, "R2_tilde_UL{k} Display"/1  "R2_tilde_UL{k}"
  "left-multiply inv(R2_tilde_UL{k}) by (C2*G2)^T "/1 -> "G2^T*C2^T*inv(R2_tilde_UL{k})"/1, "right-multiply G2^T*C2^T*inv(R2_tilde_UL{k}) by C2*G2"/1  "G2^T*C2^T*inv(R2_tilde_UL{k})"

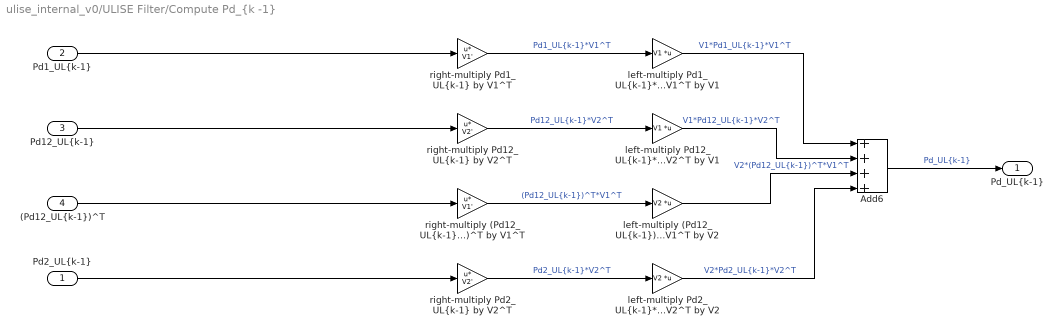
== system ulise_internal_v0/ULISE Filter/Compute Pd_{k -1} ==
  "Pd2_UL{k-1}" : Inport
  "Pd1_UL{k-1}" : Inport  Port=2
  "Pd12_UL{k-1}" : Inport  Port=3
  "(Pd12_UL{k-1})^T" : Inport  Port=4
  Add6 : Sum  Inputs=++++
  "left-multiply (Pd12_UL{k-1})^T*V1^T by V2" : Gain  Gain=V2  Multiplication=Matrix(K*u)
  "left-multiply Pd12_UL{k-1}*V2^T by V1" : Gain  Gain=V1  Multiplication=Matrix(K*u)
  "left-multiply Pd1_UL{k-1}*V1^T by V1" : Gain  Gain=V1  Multiplication=Matrix(K*u)
  "left-multiply Pd2_UL{k-1}*V2^T by V2" : Gain  Gain=V2  Multiplication=Matrix(K*u)
  "right-multiply (Pd12_UL{k-1})^T by V1^T" : Gain  Gain=V1'  Multiplication=Matrix(u*K)
  "right-multiply Pd12_UL{k-1} by V2^T" : Gain  Gain=V2'  Multiplication=Matrix(u*K)
  "right-multiply Pd1_UL{k-1} by V1^T" : Gain  Gain=V1'  Multiplication=Matrix(u*K)
  "right-multiply Pd2_UL{k-1} by V2^T" : Gain  Gain=V2'  Multiplication=Matrix(u*K)
  "Pd_UL{k-1}" : Outport
  wires:
  "Pd2_UL{k-1}"/1 -> "right-multiply Pd2_UL{k-1} by V2^T"/1
  "Pd12_UL{k-1}"/1 -> "right-multiply Pd12_UL{k-1} by V2^T"/1
  "left-multiply Pd12_UL{k-1}*V2^T by V1"/1 -> Add6/2  "V1*Pd12_UL{k-1}*V2^T"
  "Pd1_UL{k-1}"/1 -> "right-multiply Pd1_UL{k-1} by V1^T"/1
  "(Pd12_UL{k-1})^T"/1 -> "right-multiply (Pd12_UL{k-1})^T by V1^T"/1
  "left-multiply Pd2_UL{k-1}*V2^T by V2"/1 -> Add6/4  "V2*Pd2_UL{k-1}*V2^T"
  "right-multiply Pd12_UL{k-1} by V2^T"/1 -> "left-multiply Pd12_UL{k-1}*V2^T by V1"/1  "Pd12_UL{k-1}*V2^T"
  "left-multiply Pd1_UL{k-1}*V1^T by V1"/1 -> Add6/1  "V1*Pd1_UL{k-1}*V1^T"
  "right-multiply (Pd12_UL{k-1})^T by V1^T"/1 -> "left-multiply (Pd12_UL{k-1})^T*V1^T by V2"/1  "(Pd12_UL{k-1})^T*V1^T"
  Add6/1 -> "Pd_UL{k-1}"/1  "Pd_UL{k-1}"
  "right-multiply Pd1_UL{k-1} by V1^T"/1 -> "left-multiply Pd1_UL{k-1}*V1^T by V1"/1  "Pd1_UL{k-1}*V1^T"
  "right-multiply Pd2_UL{k-1} by V2^T"/1 -> "left-multiply Pd2_UL{k-1}*V2^T by V2"/1  "Pd2_UL{k-1}*V2^T"
  "left-multiply (Pd12_UL{k-1})^T*V1^T by V2"/1 -> Add6/3  "V2*(Pd12_UL{k-1})^T*V1^T"

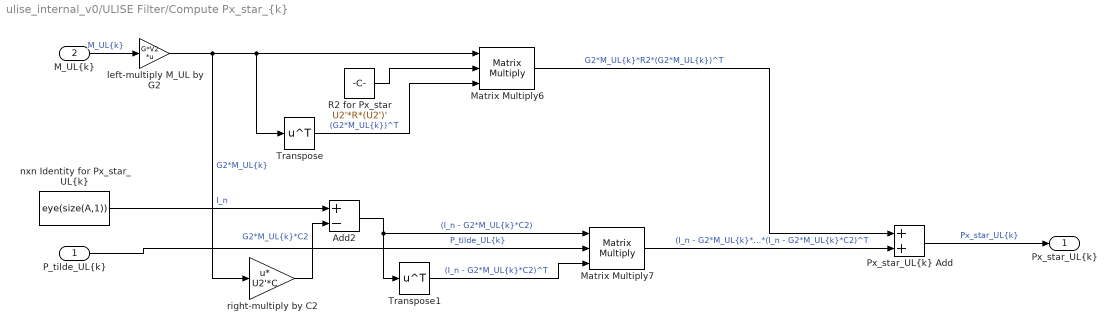
== system ulise_internal_v0/ULISE Filter/Compute Px_star_{k} ==
  "P_tilde_UL{k}" : Inport
  "M_UL{k}" : Inport  Port=2
  " R2 for Px_star" : Constant  Value=U2'*R*(U2')'
  Add2 : Sum  Inputs=+-
  Matrix Multiply6 : Product  Inputs=3  Multiplication=Matrix(*)
  Matrix Multiply7 : Product  Inputs=3  Multiplication=Matrix(*)
  "Px_star_UL{k} Add" : Sum
  Transpose : Math  Operator=transpose
  Transpose1 : Math  Operator=transpose
  left-multiply M_UL by G2 : Gain  Gain=G*V2  Multiplication=Matrix(K*u)
  "nxn Identity for Px_star_UL{k}" : Constant  Value=eye(size(A,1))  VectorParams1D=off
  right-multiply by C2 : Gain  Gain=U2'*C  Multiplication=Matrix(u*K)
  "Px_star_UL{k}" : Outport
  wires:
  right-multiply by C2/1 -> Add2/2  "G2*M_UL{k}*C2"
  left-multiply M_UL by G2/1 -> right-multiply by C2/1, Transpose/1, Matrix Multiply6/1  "G2*M_UL{k}"
  Transpose1/1 -> Matrix Multiply7/3  "(I_n - G2*M_UL{k}*C2)^T"
  Matrix Multiply7/1 -> "Px_star_UL{k} Add"/2  "(I_n - G2*M_UL{k}*C2)*P_tilde*(I_n - G2*M_UL{k}*C2)^T"
  " R2 for Px_star"/1 -> Matrix Multiply6/2
  "M_UL{k}"/1 -> left-multiply M_UL by G2/1  "M_UL{k}"
  "P_tilde_UL{k}"/1 -> Matrix Multiply7/2  "P_tilde_UL{k}"
  "Px_star_UL{k} Add"/1 -> "Px_star_UL{k}"/1  "Px_star_UL{k}"
  Add2/1 -> Matrix Multiply7/1, Transpose1/1  "(I_n - G2*M_UL{k}*C2)"
  "nxn Identity for Px_star_UL{k}"/1 -> Add2/1  "I_n"
  Transpose/1 -> Matrix Multiply6/3  "(G2*M_UL{k})^T"
  Matrix Multiply6/1 -> "Px_star_UL{k} Add"/1  "G2*M_UL{k}*R2*(G2*M_UL{k})^T"

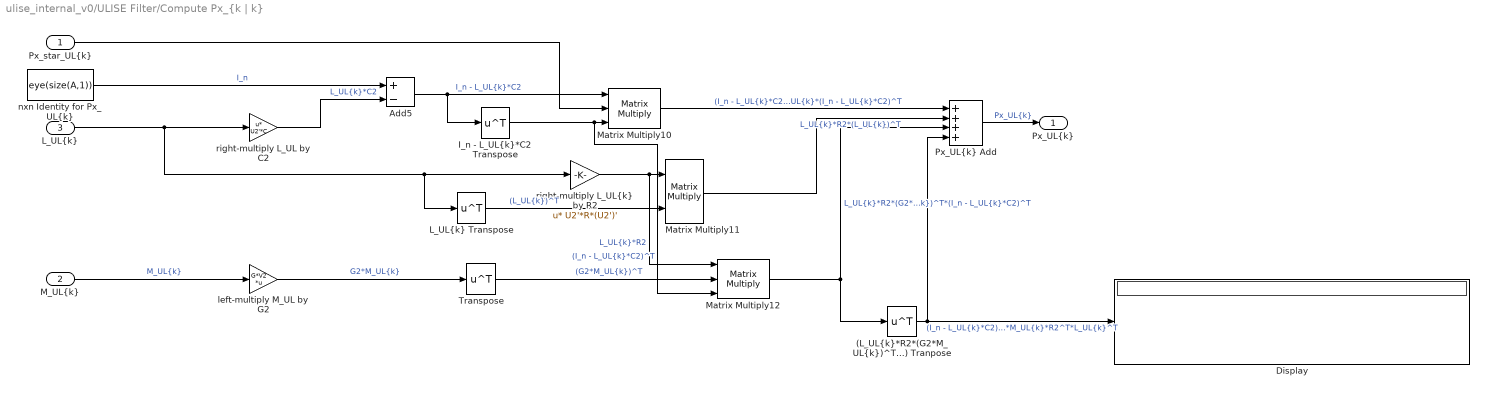
== system ulise_internal_v0/ULISE Filter/Compute Px_{k | k} ==
  "Px_star_UL{k}" : Inport
  "M_UL{k}" : Inport  Port=2
  "L_UL{k}" : Inport  Port=3
  "(L_UL{k}*R2*(G2*M_UL{k})^T*(I_n - L_UL{k}*C2)^T) Tranpose" : Math  Operator=transpose
  Add5 : Sum  Inputs=+-
  Display : Display
  "I_n - L_UL{k}*C2 Transpose" : Math  Operator=transpose
  "L_UL{k} Transpose" : Math  Operator=transpose
  Matrix Multiply10 : Product  Inputs=3  Multiplication=Matrix(*)
  Matrix Multiply11 : Product  Multiplication=Matrix(*)
  Matrix Multiply12 : Product  Inputs=3  Multiplication=Matrix(*)
  "Px_UL{k} Add" : Sum  Inputs=++++
  Transpose : Math  Operator=transpose
  left-multiply M_UL by G2 : Gain  Gain=G*V2  Multiplication=Matrix(K*u)
  "nxn Identity for Px_UL{k}" : Constant  Value=eye(size(A,1))  VectorParams1D=off
  right-multiply L_UL by C2 : Gain  Gain=U2'*C  Multiplication=Matrix(u*K)
  "right-multiply L_UL{k} by R2" : Gain  Gain=U2'*R*(U2')'  Multiplication=Matrix(u*K)
  "Px_UL{k}" : Outport
  wires:
  "Px_star_UL{k}"/1 -> Matrix Multiply10/2
  "L_UL{k} Transpose"/1 -> Matrix Multiply11/2  "(L_UL{k})^T"
  Add5/1 -> "I_n - L_UL{k}*C2 Transpose"/1, Matrix Multiply10/1  "I_n - L_UL{k}*C2"
  Matrix Multiply10/1 -> "Px_UL{k} Add"/1  "(I_n - L_UL{k}*C2)*Px_star_UL{k}*(I_n - L_UL{k}*C2)^T"
  "Px_UL{k} Add"/1 -> "Px_UL{k}"/1  "Px_UL{k}"
  Matrix Multiply12/1 -> "Px_UL{k} Add"/3, "(L_UL{k}*R2*(G2*M_UL{k})^T*(I_n - L_UL{k}*C2)^T) Tranpose"/1  "L_UL{k}*R2*(G2*M_UL{k})^T*(I_n - L_UL{k}*C2)^T"
  "(L_UL{k}*R2*(G2*M_UL{k})^T*(I_n - L_UL{k}*C2)^T) Tranpose"/1 -> Display/1, "Px_UL{k} Add"/4  "(I_n - L_UL{k}*C2)*G2*M_UL{k}*R2^T*L_UL{k}^T"
  right-multiply L_UL by C2/1 -> Add5/2  "L_UL{k}*C2"
  "L_UL{k}"/1 -> right-multiply L_UL by C2/1, "L_UL{k} Transpose"/1, "right-multiply L_UL{k} by R2"/1
  Matrix Multiply11/1 -> "Px_UL{k} Add"/2  "L_UL{k}*R2*(L_UL{k})^T"
  "right-multiply L_UL{k} by R2"/1 -> Matrix Multiply12/1, Matrix Multiply11/1  "L_UL{k}*R2"
  "nxn Identity for Px_UL{k}"/1 -> Add5/1  "I_n"
  "I_n - L_UL{k}*C2 Transpose"/1 -> Matrix Multiply12/3, Matrix Multiply10/3  "(I_n - L_UL{k}*C2)^T"
  "M_UL{k}"/1 -> left-multiply M_UL by G2/1  "M_UL{k}"
  left-multiply M_UL by G2/1 -> Transpose/1  "G2*M_UL{k}"
  Transpose/1 -> Matrix Multiply12/2  "(G2*M_UL{k})^T"

== system ulise_internal_v0/ULISE Filter/Compute Pxd1_{k} ==
  "Px_UL{k}" : Inport
  "right-multiply Px_UL{k} by -C1^T*M1^T" : Gain  Gain=-1*((U1' - U1'*R*U2*inv(U2'*R*U2)*U2')*C)'*(pinv(Sigma))'  Multiplication=Matrix(u*K)
  "Pxd1_UL{k}" : Outport
  wires:
  "Px_UL{k}"/1 -> "right-multiply Px_UL{k} by -C1^T*M1^T"/1
  "right-multiply Px_UL{k} by -C1^T*M1^T"/1 -> "Pxd1_UL{k}"/1  "Pxd1_UL{k}"

== system ulise_internal_v0/ULISE Filter/Compute measurement update, xhat_{k | k} ==
  "L_UL{k}" : Inport
  "z2{k}" : Inport  Port=2
  "xhat_star_UL{k}" : Inport  Port=3
  "u{k-1}" : Inport  Port=4
  Add3 : Sum  Inputs=+--
  Add4 : Sum
  Matrix Multiply9 : Product  Multiplication=Matrix(*)
  "left-multiply u{k} by D2" : Gain  Gain=U2'*D  Multiplication=Matrix(K*u)
  "left-multiply xhat_star_UL{k} by C2" : Gain  Gain=U2'*C  Multiplication=Matrix(K*u)
  "xhat_UL{k}" : Outport
  wires:
  "left-multiply xhat_star_UL{k} by C2"/1 -> Add3/3
  Add4/1 -> "xhat_UL{k}"/1  "xhat_UL{k}"
  "z2{k}"/1 -> Add3/1
  "xhat_star_UL{k}"/1 -> "left-multiply xhat_star_UL{k} by C2"/1, Add4/1
  Matrix Multiply9/1 -> Add4/2  "L_ULk}*(z2{k} - D2*u{k} - C2*xhat_star_UL{k})"
  "u{k-1}"/1 -> "left-multiply u{k} by D2"/1
  "left-multiply u{k} by D2"/1 -> Add3/2  "D2*u{k}"
  "L_UL{k}"/1 -> Matrix Multiply9/1
  Add3/1 -> Matrix Multiply9/2  "z2{k} - D2*u{k} - C2*xhat_star_UL{k}"

== system ulise_internal_v0/ULISE Filter/Compute observable unknown input, dhat1_{k} ==
  "z1{k}" : Inport
  "xhat_UL{k}" : Inport  Port=2
  "u{k-1}" : Inport  Port=3
  dhat1 Add block : Sum  Inputs=+--
  left-multiply by M1 : Gain  Gain=pinv(Sigma)  Multiplication=Matrix(K*u)
  "left-multiply u{k} by D1" : Gain  Gain=(U1' - U1'*R*U2*inv(U2'*R*U2)*U2')*D  Multiplication=Matrix(K*u)
  "left-multiply xhat_UL{k} by C1" : Gain  Gain=(U1' - U1'*R*U2*inv(U2'*R*U2)*U2')*C  Multiplication=Matrix(K*u)
  "dhat1_UL{k}" : Outport
  wires:
  "xhat_UL{k}"/1 -> "left-multiply xhat_UL{k} by C1"/1
  left-multiply by M1/1 -> "dhat1_UL{k}"/1  "dhat1_UL{k}"
  "left-multiply u{k} by D1"/1 -> dhat1 Add block/3
  "left-multiply xhat_UL{k} by C1"/1 -> dhat1 Add block/2
  "z1{k}"/1 -> dhat1 Add block/1  "z1{k}"
  "u{k-1}"/1 -> "left-multiply u{k} by D1"/1
  dhat1 Add block/1 -> left-multiply by M1/1  "z1{k} - C1*xhat_UL{k} - D1*u{k}"

== system ulise_internal_v0/ULISE Filter/Compute state prediction, xhat_{k | k-1}  ==
  note: state estimate at current time step
  "xhat_UL{k-1}" : Inport
  "u{k-1}" : Inport  Port=2
  "dhat1_UL{k-1}" : Inport  Port=3
  left-multiply by A : Gain  Gain=A  Multiplication=Matrix(K*u)
  left-multiply by B : Gain  Gain=B  Multiplication=Matrix(K*u)
  left-multiply by G : Gain  Gain=G*V1  Multiplication=Matrix(K*u)
  "xhat_p_UL{k} Add" : Sum  Inputs=+++
  "xhat_p_UL{k}" : Outport
  wires:
  "dhat1_UL{k-1}"/1 -> left-multiply by G/1
  left-multiply by B/1 -> "xhat_p_UL{k} Add"/2  "B*u{k-1}"
  left-multiply by A/1 -> "xhat_p_UL{k} Add"/1  "A*xhat_UL{k-1}"
  "u{k-1}"/1 -> left-multiply by B/1
  "xhat_p_UL{k} Add"/1 -> "xhat_p_UL{k}"/1  "xhat_p_UL{k}"
  "xhat_UL{k-1}"/1 -> left-multiply by A/1
  left-multiply by G/1 -> "xhat_p_UL{k} Add"/3  "G*dhat1_UL{k-1}"

== system ulise_internal_v0/ULISE Filter/Compute time updated state, xhat_star_{k | k} ==
  "xhat_p_UL{k}" : Inport
  "dhat2_UL{k-1}" : Inport  Port=2
  left-multiply by G2 : Gain  Gain=G*V2  Multiplication=Matrix(K*u)
  "xhat_star_UL{k} Add" : Sum
  "xhat_star_UL{k}" : Outport
  wires:
  "dhat2_UL{k-1}"/1 -> left-multiply by G2/1
  "xhat_p_UL{k}"/1 -> "xhat_star_UL{k} Add"/1
  "xhat_star_UL{k} Add"/1 -> "xhat_star_UL{k}"/1  "xhat_star_UL{k}"
  left-multiply by G2/1 -> "xhat_star_UL{k} Add"/2  "G2*dhat2_UL{k-1}"

== system ulise_internal_v0/ULISE Filter/Compute unknown input, dhat_{k-1} ==
  "dhat1_UL{k-1}" : Inport
  "dhat2_UL{k-1}" : Inport  Port=2
  "dhat_UL{k-1} Mux" : Mux  Inputs=2
  left-multiply by V : Gain  Gain=V  Multiplication=Matrix(K*u)
  "dhat_UL{k-1}" : Outport
  wires:
  "dhat2_UL{k-1}"/1 -> "dhat_UL{k-1} Mux"/2
  "dhat1_UL{k-1}"/1 -> "dhat_UL{k-1} Mux"/1
  left-multiply by V/1 -> "dhat_UL{k-1}"/1  "dhat_UL{k-1}"
  "dhat_UL{k-1} Mux"/1 -> left-multiply by V/1  "[dhat1{k-1}; dhat2{k-1}]"

== system ulise_internal_v0/ULISE Filter/Compute unobservable unknown input, dhat2_{k-1} ==
  note: unknown unobservable input estimate at previous time step
  "M_UL{k}" : Inport
  "xhat_p_UL{k}" : Inport  Port=2
  "z2{k}" : Inport  Port=3
  "u{k-1}" : Inport  Port=4
  Matrix Multiply1 : Product  Multiplication=Matrix(*)
  dhat2 Add/Sub block : Sum  Inputs=+--
  left-multiply by C2_dhat2 : Gain  Gain=U2'*C  Multiplication=Matrix(K*u)
  left-multiply by D2 : Gain  Gain=U2'*D  Multiplication=Matrix(K*u)
  "dhat2_UL{k-1}" : Outport
  wires:
  "M_UL{k}"/1 -> Matrix Multiply1/1
  dhat2 Add/Sub block/1 -> Matrix Multiply1/2  "dhat2_UL{k-1}"
  "u{k-1}"/1 -> left-multiply by D2/1
  "z2{k}"/1 -> dhat2 Add/Sub block/1
  left-multiply by C2_dhat2/1 -> dhat2 Add/Sub block/2  "C2*xhat_p_UL{k}"
  left-multiply by D2/1 -> dhat2 Add/Sub block/3  "D2*u{k-1}"
  Matrix Multiply1/1 -> "dhat2_UL{k-1}"/1  "dhat2_UL{k-1}"
  "xhat_p_UL{k}"/1 -> left-multiply by C2_dhat2/1

== matlab function ulise_internal_v0/MATLAB Function ==
  data: A input; y output
function y = fcn(A)

y1 = svd(A,"economy");
y_inv = 
y2 = inv(A'*A)*A';
y3 = A'*inv(A*A');

y = u;
